simulink model "cf_compare_model"  (R2016a)
settings: Solver=FixedStepAuto  StartTime=0.0  StopTime=50  FixedStep=dt  RelTol=1e-3
values from neighbouring files (symbols this model uses):
  circ_amp = 3    [cf_pid_compare.m]
  circ_w = k    (= 0.666666666667)    [cf_pid_compare.m]
  ic = [-3 0 0 0 0 0 0 0 0 0 0 0]    [cf_pid_compare.m]    (also in main.m = [0 0 0 0 0 0 0 0 0 0 0 0])
  r2d = 180/pi    (= 57.2957795131)    [main.m]
  x_init = 0.0    (= 0)    [cf_pid_compare.m]
  x_vel = 1.0    (= 1)    [cf_pid_compare.m]
undefined symbols (not defined in the file or in its folder): default_ctl, est, geometric_ctl, pid_ctl
undefined symbols (not defined in the file): cf2
libraries: simulink x18, vrlib x12, aerolibtransform2 x12, cstblocks x8, aerolibutil x6, aerolibnav x3, dspmathops x2
(part 1 of 2)
settings Model: Creator=appatte2  LastModifiedBy=arun
settings DebuggingCC: SFUnusedDataAndEventsDiag=none

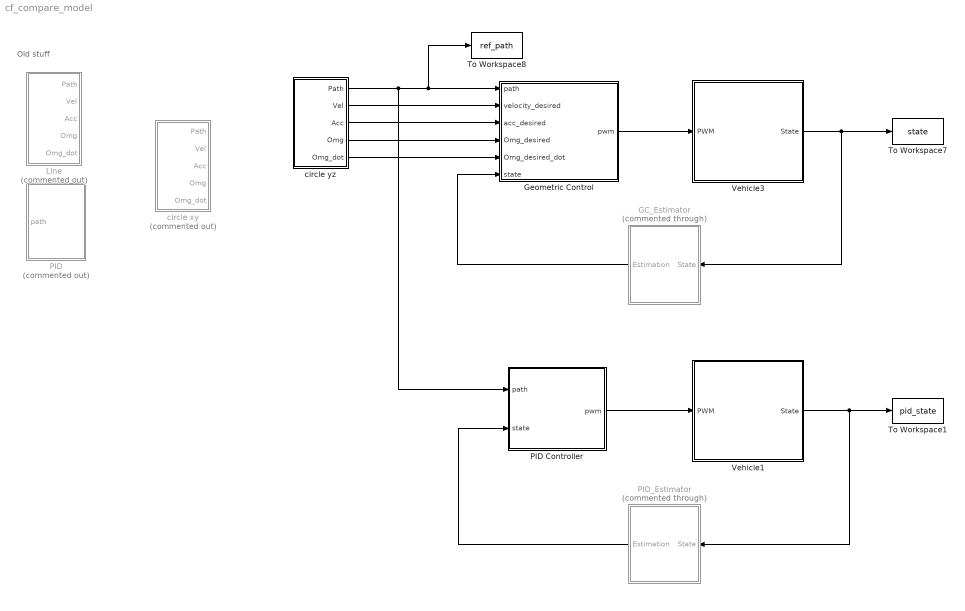
== system cf_compare_model ==
  note: Old stuff
  GC_Estimator : Subsystem  Commented=through  mask{rng_seed=1111, est=est}
      mask prompts: rng_seed "Random Seed"; est "Estimator Params"
  Geometric Control : Subsystem  mask(PID Controller for Quadrotor){model=cf2, ctl=geometric_ctl}
      mask prompts: model "Quad Model"; ctl "Controller"
      mask help: Allows user to set parameters for pid controllers on rates, angles and linear position.
  Line : Subsystem  Commented=on
  PID : Subsystem  Commented=on
  PID Controller : Subsystem  mask(PID Controller for Quadrotor){mix=pid_ctl.mix, rates=pid_ctl.rates, att=pid_ctl.att, pos=pid_ctl.pos, sat=pid_ctl.sat, intSat=pid_ctl.intSat}
      mask prompts: mix "Motor Mixing Table"; rates "Rate Control Table"; att "Attitude Control Table"; pos "Position Control Table"; sat "Attitude Limits"; intSat "Integral Saturation"
      mask help: Allows user to set parameters for pid controllers on rates, angles and linear position.
  PID_Estimator : Subsystem  Commented=through  mask{rng_seed=1111, est=est}
      mask prompts: rng_seed "Random Seed"; est "Estimator Params"
  To Workspace1 : ToWorkspace  VariableName=pid_state  SampleTime=-1
  To Workspace7 : ToWorkspace  VariableName=state  SampleTime=-1
  To Workspace8 : ToWorkspace  VariableName=ref_path  SampleTime=-1
      settings: Save2DSignal=2-D array (concatenate along first dimension)
  Vehicle1 : Subsystem  mask{model=cf2, ic=ic}
      mask prompts: model "Model Object"; ic "Initial Condition"
  Vehicle3 : Subsystem  mask{model=cf2, ic=ic}
      mask prompts: model "Model Object"; ic "Initial Condition"
  circle xy : Subsystem  Commented=on
  "circle yz " : Subsystem
  wires:
  "circle yz "/1(Path) -> PID Controller/1(path), Geometric Control/1(path), To Workspace8/1
  "circle yz "/2(Vel) -> Geometric Control/2(velocity_desired)
  "circle yz "/3(Acc) -> Geometric Control/3("acc_desired ")
  "circle yz "/4(Omg) -> Geometric Control/4(Omg_desired)
  "circle yz "/5(Omg_dot) -> Geometric Control/5(Omg_desired_dot)
  GC_Estimator/1(Estimation) -> Geometric Control/6(state)
  Geometric Control/1(pwm) -> Vehicle3/1(PWM)
  Vehicle3/1(State) -> GC_Estimator/1(State), To Workspace7/1
  PID Controller/1(pwm) -> Vehicle1/1(PWM)
  Vehicle1/1(State) -> PID_Estimator/1(State), To Workspace1/1
  PID_Estimator/1(Estimation) -> PID Controller/2(state)

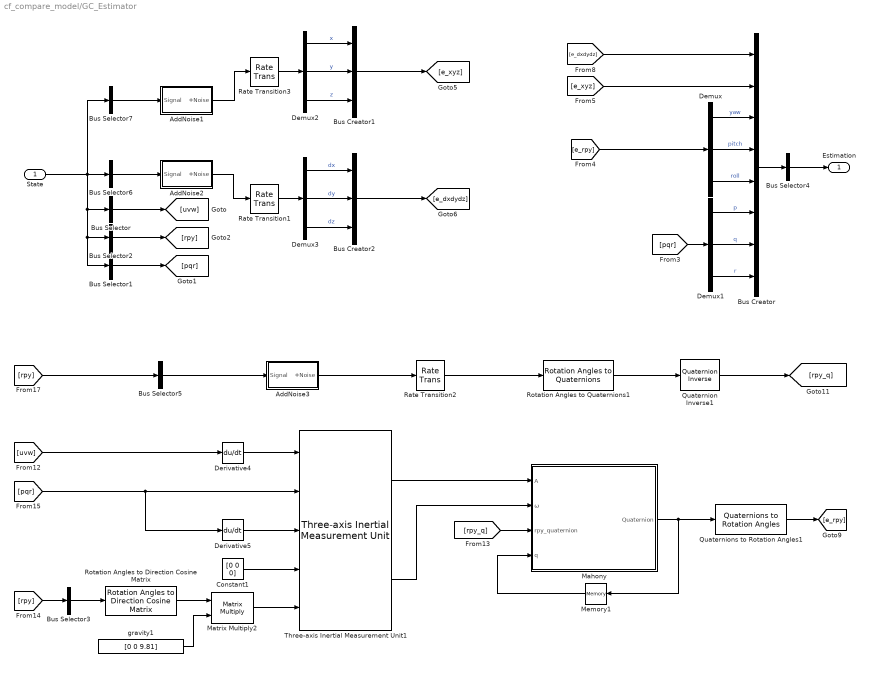
== system cf_compare_model/GC_Estimator ==
  State : Inport
  AddNoise1 : Subsystem
  AddNoise2 : Subsystem
  AddNoise3 : Subsystem
  Bus Creator : BusCreator  Inputs=8
  Bus Creator1 : BusCreator  Inputs=3
  Bus Creator2 : BusCreator  Inputs=3
  Bus Selector : BusSelector  OutputSignals=u,v,w  OutputAsBus=on
  Bus Selector1 : BusSelector  OutputSignals=p,q,r  OutputAsBus=on
  Bus Selector2 : BusSelector  OutputSignals=roll,pitch,yaw  OutputAsBus=on
  Bus Selector3 : BusSelector  OutputSignals=yaw,pitch,roll  OutputAsBus=on
  Bus Selector4 : BusSelector  OutputSignals=signal2.x,signal2.y,signal2.z,signal1.dx,signal1.dy,signal1.dz,roll,pitch,yaw,p,q,r  OutputAsBus=on
  Bus Selector5 : BusSelector  OutputSignals=yaw,pitch,roll  OutputAsBus=on
  Bus Selector6 : BusSelector  OutputSignals=dx,dy,dz  OutputAsBus=on
  Bus Selector7 : BusSelector  OutputSignals=x,y,z  OutputAsBus=on
  Constant1 : Constant  Value=[0 0 0]
  Demux{,1..3} (4 alike) : Demux  Outputs=3
  Derivative4 : Derivative
  Derivative5 : Derivative
  Mahony : Subsystem
  Matrix Multiply2 : Product  Multiplication=Matrix(*)
  Memory1 : Memory  X0=[1 0 0 0]
  Quaternion Inverse1 : aerolibutil/Quaternion Inverse
  Quaternions to Rotation Angles1 : aerolibtransform2/Quaternions to Rotation Angles  rotationOrder=ZYX
  Rate Transition1 : RateTransition  OutPortSampleTime=0.004
  Rate Transition2 : RateTransition  OutPortSampleTime=0.004
  Rate Transition3 : RateTransition  OutPortSampleTime=0.004
  Rotation Angles to Direction Cosine Matrix : aerolibtransform2/Rotation Angles to Direction Cosine Matrix  rotationOrder=ZYX
  Rotation Angles to Quaternions1 : aerolibtransform2/Rotation Angles to Quaternions  rotationOrder=ZYX
  Three-axis Inertial Measurement Unit1 : aerolibnav/Three-axis Inertial Measurement Unit  units=Metric (MKS)  imu=[0 0 0]  dtype_a=on  w_a=190  z_a=0.707  a_sf_cc=[0.98 0 0; 0 0.98 0; 0 0 0.98]  a_bias=[0 0 0]  a_sat="[-19.62  -19.62  -19.62 19.62 19.62 19.62]"  dtype_g=on  w_g=190  z_g=0.707  g_sf_cc=[.98 0 0; 0 .98 0; 0 0 .98]  g_bias=[0 0 0]  g_sens=[0 0 0]  g_sat="[-4.36  -4.36  -4.36 4.36 4.36 4.36]"  i_rand=on  i_seeds=[23093 23094 23095 23096 23097 23098]*rng_seed  i_pow=[0.001 0.001 0.001 0.0001 0.0001 0.0001]*10  i_Ts=0
  gravity1 : Constant  Value=[0 0 9.81]
  Estimation : Outport
  wires:
  Bus Creator2/1 -> [e_dxdydz]
  Demux3/1 -> Bus Creator2/1  "dx"
  Demux3/2 -> Bus Creator2/2  "dy"
  Demux3/3 -> Bus Creator2/3  "dz"
  Bus Creator1/1 -> [e_xyz]
  Demux2/2 -> Bus Creator1/2  "y"
  Demux2/3 -> Bus Creator1/3  "z"
  Demux2/1 -> Bus Creator1/1  "x"
  Bus Selector4/1 -> Estimation/1
  Demux/3 -> Bus Creator/5  "roll"
  Demux/1 -> Bus Creator/3  "yaw"
  Demux/2 -> Bus Creator/4  "pitch"
  Bus Selector2/1 -> [rpy]
  Bus Selector1/1 -> [pqr]
  Bus Selector/1 -> [uvw]
  Bus Creator/1 -> Bus Selector4/1
  State/1 -> Bus Selector6/1, Bus Selector/1, Bus Selector2/1, Bus Selector1/1, Bus Selector7/1
  Demux1/1 -> Bus Creator/6  "p"
  Demux1/2 -> Bus Creator/7  "q"
  [pqr] -> Demux1/1
  Demux1/3 -> Bus Creator/8  "r"
  Quaternions to Rotation Angles1/1 -> [e_rpy]
  [rpy] -> Bus Selector5/1
  AddNoise3/1(+Noise) -> Rate Transition2/1
  Rate Transition2/1 -> Rotation Angles to Quaternions1/1
  [rpy_q] -> Mahony/3(rpy_quaternion)
  Rotation Angles to Quaternions1/1 -> Quaternion Inverse1/1
  [rpy] -> Bus Selector3/1
  [pqr] -> Derivative5/1, Three-axis Inertial Measurement Unit1/2
  [uvw] -> Derivative4/1
  Matrix Multiply2/1 -> Three-axis Inertial Measurement Unit1/5
  Rotation Angles to Direction Cosine Matrix/1 -> Matrix Multiply2/1
  gravity1/1 -> Matrix Multiply2/2
  Derivative5/1 -> Three-axis Inertial Measurement Unit1/3
  Three-axis Inertial Measurement Unit1/2 -> Mahony/2(ω)
  Three-axis Inertial Measurement Unit1/1 -> Mahony/1(A)
  Mahony/1(Quaternion) -> Quaternions to Rotation Angles1/1, Memory1/1
  Memory1/1 -> Mahony/4(q)
  Constant1/1 -> Three-axis Inertial Measurement Unit1/4
  Derivative4/1 -> Three-axis Inertial Measurement Unit1/1
  Bus Selector3/1 -> Rotation Angles to Direction Cosine Matrix/1
  Quaternion Inverse1/1 -> [rpy_q]
  Bus Selector5/1 -> AddNoise3/1(Signal)
  Bus Selector6/1 -> AddNoise2/1(Signal)
  AddNoise1/1(+Noise) -> Rate Transition3/1
  Bus Selector7/1 -> AddNoise1/1(Signal)
  Rate Transition1/1 -> Demux3/1
  Rate Transition3/1 -> Demux2/1
  AddNoise2/1(+Noise) -> Rate Transition1/1
  [e_rpy] -> Demux/1
  [e_dxdydz] -> Bus Creator/1
  [e_xyz] -> Bus Creator/2

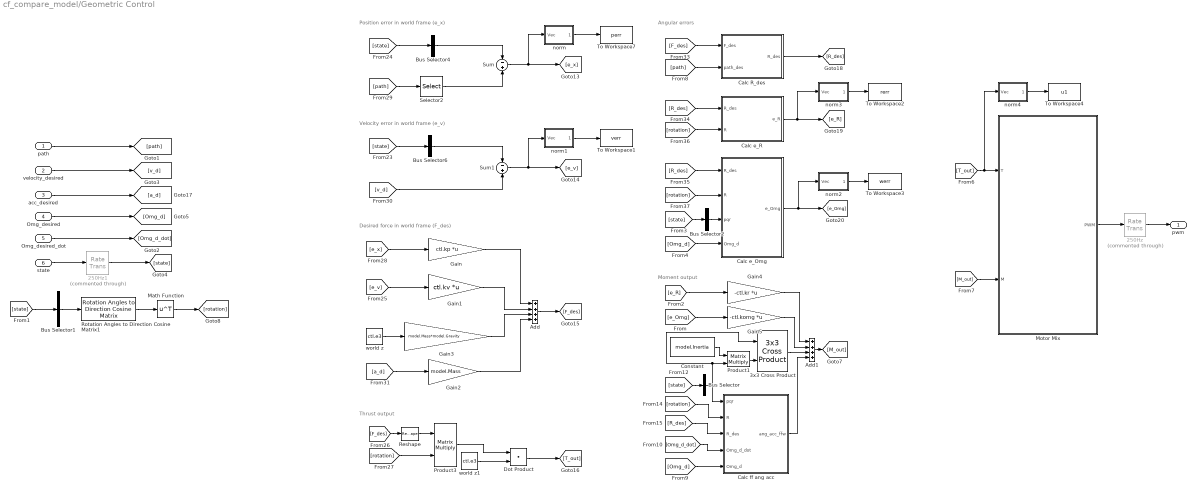
== system cf_compare_model/Geometric Control ==
  note: Moment output
  note: Angular errors
  note: Thrust output
  note: Desired force in world frame (F_des)
  note: Velocity error in world frame (e_v)
  note: Position error in world frame (e_x)
  path : Inport
  velocity_desired : Inport  Port=2
  "acc_desired " : Inport  Port=3
  Omg_desired : Inport  Port=4
  Omg_desired_dot : Inport  Port=5
  state : Inport  Port=6
  250Hz : RateTransition  Commented=through  OutPortSampleTime=0.004
  250Hz1 : RateTransition  Commented=through  OutPortSampleTime=0.004
  3x3 Cross Product : aerolibutil/3x3 Cross Product
  Add : Sum  Inputs=++++
  Add1 : Sum  Inputs=++++
  Bus Selector : BusSelector  OutputSignals=p,q,r  OutputAsBus=on
  Bus Selector1 : BusSelector  OutputSignals=yaw,pitch,roll  OutputAsBus=on
  Bus Selector2 : BusSelector  OutputSignals=p,q,r  OutputAsBus=on
  Bus Selector4 : BusSelector  OutputSignals=x,y,z  OutputAsBus=on
  Bus Selector6 : BusSelector  OutputSignals=dx,dy,dz  OutputAsBus=on
  Calc R_des : Subsystem
  Calc e_Omg : Subsystem
  Calc e_R : Subsystem
  Calc ff ang acc : Subsystem
  Constant : Constant  Value=model.Inertia
  Dot Product : DotProduct  InputSameDT=on  OutDataTypeStr=Inherit: Inherit via internal rule
  Gain : Gain  Gain=ctl.kp  Multiplication=Matrix(K*u) (u vector)
  Gain1 : Gain  Gain=ctl.kv  Multiplication=Matrix(K*u) (u vector)
  Gain2 : Gain  Gain=model.Mass
  Gain3 : Gain  Gain=model.Mass*model.Gravity
  Gain4 : Gain  Gain=-ctl.kr  Multiplication=Matrix(K*u) (u vector)
  Gain5 : Gain  Gain=-ctl.komg  Multiplication=Matrix(K*u) (u vector)
  Math Function : Math  Operator=transpose  SaturateOnIntegerOverflow=on
  Motor Mix : Subsystem
  Product1 : Product  Multiplication=Matrix(*)
  Product3 : Product  Multiplication=Matrix(*)
  Reshape : Reshape  OutputDimensionality=Row vector (2-D)
  Rotation Angles to Direction Cosine Matrix1 : aerolibtransform2/Rotation Angles to Direction Cosine Matrix  rotationOrder=ZYX
  Selector2 : Selector  InputPortWidth=4  IndexOptions=Index vector (dialog)  Indices=[1 2 3]  OutputSizes=1
  Sum : Sum  Inputs=-|+
  Sum1 : Sum  Inputs=-|+
  To Workspace1 : ToWorkspace  VariableName=verr  SaveFormat=Timeseries  SampleTime=-1
  To Workspace2 : ToWorkspace  VariableName=rerr  SaveFormat=Timeseries  SampleTime=-1
  To Workspace3 : ToWorkspace  VariableName=werr  SaveFormat=Timeseries  SampleTime=-1
  To Workspace4 : ToWorkspace  VariableName=u1  SaveFormat=Timeseries  SampleTime=-1
  To Workspace7 : ToWorkspace  VariableName=perr  SaveFormat=Timeseries  SampleTime=-1
  norm : Subsystem
  norm1 : Subsystem
  norm2 : Subsystem
  norm3 : Subsystem
  norm4 : Subsystem
  world z : Constant  Value=ctl.e3
  world z1 : Constant  Value=ctl.e3
  pwm : Outport
  wires:
  state/1 -> 250Hz1/1
  path/1 -> [path]
  velocity_desired/1 -> [v_d]
  Motor Mix/1(PWM) -> 250Hz/1
  [path] -> Selector2/1
  [state] -> Bus Selector4/1
  Bus Selector4/1 -> Sum/1
  [state] -> Bus Selector6/1
  Sum1/1 -> norm1/1(Vec), [e_v]
  [v_d] -> Sum1/2
  [e_x] -> Gain/1
  [e_v] -> Gain1/1
  [a_d] -> Gain2/1
  world z/1 -> Gain3/1
  Gain3/1 -> Add/3
  Gain2/1 -> Add/4
  Gain1/1 -> Add/2
  Gain/1 -> Add/1
  Add/1 -> [F_des]
  [F_des] -> Reshape/1
  Product3/1 -> Dot Product/1
  "acc_desired "/1 -> [a_d]
  [F_des] -> Calc R_des/1(F_des)
  [path] -> Calc R_des/2(path_des)
  Calc R_des/1(R_des) -> [R_des]
  [R_des] -> Calc e_R/1(R_des)
  [rotation] -> Calc e_R/2(R)
  Calc e_R/1(e_R) -> norm3/1(Vec), [e_R]
  [R_des] -> Calc e_Omg/1(R_des)
  [rotation] -> Calc e_Omg/2(R)
  Calc e_Omg/1(e_Omg) -> norm2/1(Vec), [e_Omg]
  Omg_desired/1 -> [Omg_d]
  [state] -> Bus Selector2/1
  [Omg_d] -> Calc e_Omg/4(Omg_d)
  Constant/1 -> Product1/1
  Product1/1 -> 3x3 Cross Product/2
  [e_R] -> Gain4/1
  [e_Omg] -> Gain5/1
  Gain4/1 -> Add1/1
  Gain5/1 -> Add1/2
  [T_out] -> norm4/1(Vec), Motor Mix/1(T)
  [M_out] -> Motor Mix/2(M)
  Sum/1 -> norm/1(Vec), [e_x]
  Selector2/1 -> Sum/2
  Dot Product/1 -> [T_out]
  [rotation] -> Product3/2
  world z1/1 -> Dot Product/2
  Reshape/1 -> Product3/1
  Bus Selector6/1 -> Sum1/1
  Add1/1 -> [M_out]
  Rotation Angles to Direction Cosine Matrix1/1 -> Math Function/1
  Math Function/1 -> [rotation]
  Bus Selector1/1 -> Rotation Angles to Direction Cosine Matrix1/1
  [state] -> Bus Selector1/1
  Omg_desired_dot/1 -> [Omg_d_dot]
  [rotation] -> Calc ff ang acc/2(R)
  [Omg_d_dot] -> Calc ff ang acc/4(Omg_d_dot)
  [Omg_d] -> Calc ff ang acc/5(Omg_d)
  [R_des] -> Calc ff ang acc/3(R_des)
  [state] -> Bus Selector/1
  Bus Selector/1 -> 3x3 Cross Product/1, Product1/2, Calc ff ang acc/1(pqr)
  Bus Selector2/1 -> Calc e_Omg/3(pqr)
  3x3 Cross Product/1 -> Add1/3
  Calc ff ang acc/1(ang_acc_ffw) -> Add1/4
  250Hz/1 -> pwm/1
  250Hz1/1 -> [state]
  norm/1(Norm) -> To Workspace7/1
  norm1/1(Norm) -> To Workspace1/1
  norm2/1(Norm) -> To Workspace3/1
  norm3/1(Norm) -> To Workspace2/1
  norm4/1(Norm) -> To Workspace4/1

== system cf_compare_model/Line ==
  note: X
      | Y
      | Z
      | Yaw
  Constant : Constant  Value=10
  Constant1 : Constant  Commented=on  Value=[2,2,0]'
  Constant2 : Constant  Commented=on  Value=[0,0,0]'
  Constant3 : Constant  Commented=on  Value=[0,0,0]'
  Constant4 : Constant  Commented=on  Value=[0,0,0]'
  Constant5 : Constant  Value=pi/4
  Gain : Gain  Commented=through  Gain=0
  Gain1 : Gain  Commented=through  Gain=0
  Mux : Mux
  Ramp : simulink/Sources/Ramp  slope=2  start=0  X0=0
  Ramp1 : simulink/Sources/Ramp  slope=2  start=0  X0=0
  Path : Outport
  Vel : Outport  Port=2
  Acc : Outport  Port=3
  Omg : Outport  Port=4
  Omg_dot : Outport  Port=5
  wires:
  Mux/1 -> Path/1
  Constant5/1 -> Mux/4
  Constant/1 -> Mux/3
  Ramp/1 -> Gain1/1
  Ramp1/1 -> Gain/1
  Gain/1 -> Mux/2
  Gain1/1 -> Mux/1
  Constant1/1 -> Vel/1
  Constant2/1 -> Acc/1
  Constant3/1 -> Omg/1
  Constant4/1 -> Omg_dot/1

== system cf_compare_model/PID ==
  path : Inport
  Estimator : Subsystem  mask{rng_seed=1111, est=est}
      mask prompts: rng_seed "Random Seed"; est "Estimator params"
  PID Controller : Subsystem  mask(PID Controller for Quadrotor){mix=pid_ctl.mix, rates=pid_ctl.rates, att=pid_ctl.att, pos=pid_ctl.pos, sat=pid_ctl.sat, intSat=pid_ctl.intSat}
      mask prompts: mix "Motor Mixing Table"; rates "Rate Control Table"; att "Attitude Control Table"; pos "Position Control Table"; sat "Attitude Limits"; intSat "Integral Saturation"
      mask help: Allows user to set parameters for pid controllers on rates, angles and linear position.
  To Workspace1 : ToWorkspace  VariableName=pid_state  SampleTime=-1
  Vehicle : Subsystem  mask{model=cf2, ic=ic}
      mask prompts: model "Model Object"; ic "Initial Condition"
  wires:
  path/1 -> PID Controller/1(path)
  PID Controller/1(pwm) -> Vehicle/1(PWM)
  Estimator/1(Estimation) -> PID Controller/2(state)
  Vehicle/1(State) -> Estimator/1(State), To Workspace1/1

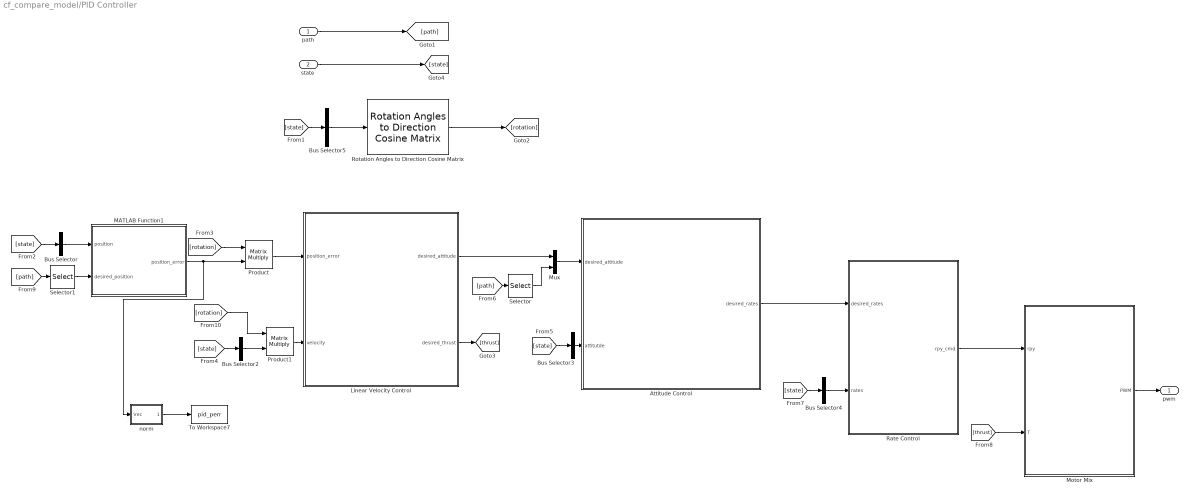
== system cf_compare_model/PID Controller ==
  path : Inport
  state : Inport  Port=2
  Attitude Control : Subsystem
  Bus Selector : BusSelector  OutputSignals=x,y,z  OutputAsBus=on
  Bus Selector2 : BusSelector  OutputSignals=dx,dy,dz  OutputAsBus=on
  Bus Selector3 : BusSelector  OutputSignals=roll,pitch,yaw  OutputAsBus=on
  Bus Selector4 : BusSelector  OutputSignals=p,q,r  OutputAsBus=on
  Bus Selector5 : BusSelector  OutputSignals=yaw,pitch,roll  OutputAsBus=on
  Linear Velocity Control : Subsystem
  MATLAB Function1 : MATLAB Function  TreatAsAtomicUnit=on
  Motor Mix : Subsystem
  Mux : Mux  Inputs=2
  Product : Product  Multiplication=Matrix(*)
  Product1 : Product  Multiplication=Matrix(*)
  Rate Control : Subsystem
  Rotation Angles to Direction Cosine Matrix : aerolibtransform2/Rotation Angles to Direction Cosine Matrix  rotationOrder=ZYX
  Selector : Selector  InputPortWidth=4  IndexOptions=Index vector (dialog)  Indices=[4]  OutputSizes=1
  Selector1 : Selector  InputPortWidth=4  IndexOptions=Index vector (dialog)  Indices=[1 2 3]  OutputSizes=1
  To Workspace7 : ToWorkspace  VariableName=pid_perr  SaveFormat=Timeseries  SampleTime=-1
  norm : Subsystem
  pwm : Outport
  wires:
  [path] -> Selector1/1
  [state] -> Bus Selector/1
  Motor Mix/1(PWM) -> pwm/1
  Selector1/1 -> MATLAB Function1/2(desired_position)
  Bus Selector/1 -> MATLAB Function1/1(position)
  [rotation] -> Product/1
  Mux/1 -> Attitude Control/1(desired_attitude)
  Bus Selector5/1 -> Rotation Angles to Direction Cosine Matrix/1
  [state] -> Bus Selector3/1
  Bus Selector3/1 -> Attitude Control/2(attitutde)
  [state] -> Bus Selector2/1
  [state] -> Bus Selector5/1
  [thrust] -> Motor Mix/2(T)
  Attitude Control/1(desired_rates) -> Rate Control/1(desired_rates)
  [state] -> Bus Selector4/1
  Bus Selector4/1 -> Rate Control/2(rates)
  [path] -> Selector/1
  Selector/1 -> Mux/2
  Linear Velocity Control/2(desired_thrust) -> [thrust]
  state/1 -> [state]
  path/1 -> [path]
  MATLAB Function1/1(position_error) -> norm/1(Vec), Product/2
  Product/1 -> Linear Velocity Control/1(position_error)
  Linear Velocity Control/1(desired_attitude) -> Mux/1
  Rotation Angles to Direction Cosine Matrix/1 -> [rotation]
  Rate Control/1(rpy_cmd) -> Motor Mix/1(rpy)
  Product1/1 -> Linear Velocity Control/2(velocity)
  Bus Selector2/1 -> Product1/2
  [rotation] -> Product1/1
  norm/1(Norm) -> To Workspace7/1

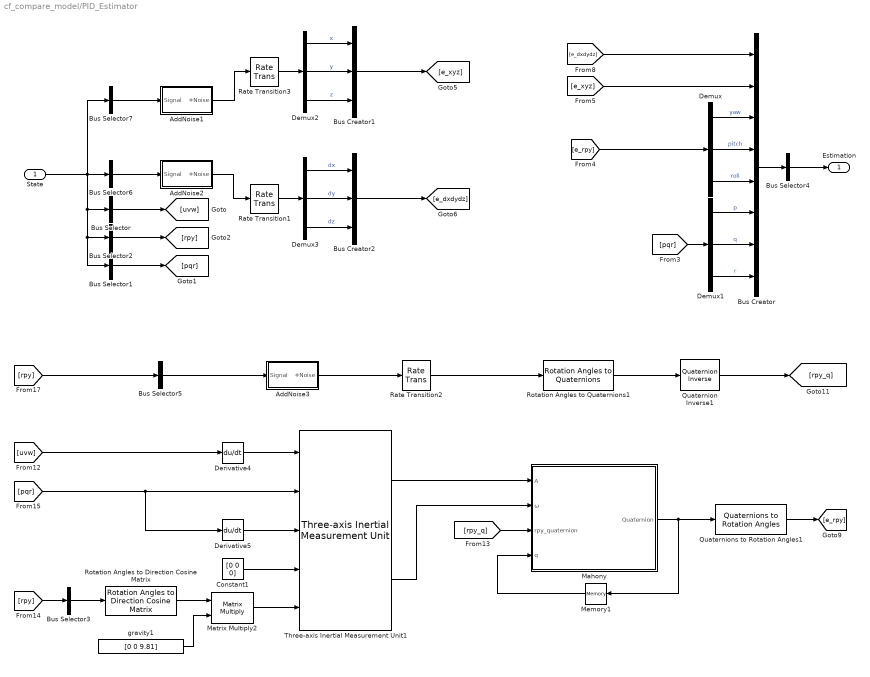
== system cf_compare_model/PID_Estimator ==
  State : Inport
  AddNoise1 : Subsystem
  AddNoise2 : Subsystem
  AddNoise3 : Subsystem
  Bus Creator : BusCreator  Inputs=8
  Bus Creator1 : BusCreator  Inputs=3
  Bus Creator2 : BusCreator  Inputs=3
  Bus Selector : BusSelector  OutputSignals=u,v,w  OutputAsBus=on
  Bus Selector1 : BusSelector  OutputSignals=p,q,r  OutputAsBus=on
  Bus Selector2 : BusSelector  OutputSignals=roll,pitch,yaw  OutputAsBus=on
  Bus Selector3 : BusSelector  OutputSignals=yaw,pitch,roll  OutputAsBus=on
  Bus Selector4 : BusSelector  OutputSignals=signal2.x,signal2.y,signal2.z,signal1.dx,signal1.dy,signal1.dz,roll,pitch,yaw,p,q,r  OutputAsBus=on
  Bus Selector5 : BusSelector  OutputSignals=yaw,pitch,roll  OutputAsBus=on
  Bus Selector6 : BusSelector  OutputSignals=dx,dy,dz  OutputAsBus=on
  Bus Selector7 : BusSelector  OutputSignals=x,y,z  OutputAsBus=on
  Constant1 : Constant  Value=[0 0 0]
  Demux{,1..3} (4 alike) : Demux  Outputs=3
  Derivative4 : Derivative
  Derivative5 : Derivative
  Mahony : Subsystem
  Matrix Multiply2 : Product  Multiplication=Matrix(*)
  Memory1 : Memory  X0=[1 0 0 0]
  Quaternion Inverse1 : aerolibutil/Quaternion Inverse
  Quaternions to Rotation Angles1 : aerolibtransform2/Quaternions to Rotation Angles  rotationOrder=ZYX
  Rate Transition1 : RateTransition  OutPortSampleTime=0.004
  Rate Transition2 : RateTransition  OutPortSampleTime=0.004
  Rate Transition3 : RateTransition  OutPortSampleTime=0.004
  Rotation Angles to Direction Cosine Matrix : aerolibtransform2/Rotation Angles to Direction Cosine Matrix  rotationOrder=ZYX
  Rotation Angles to Quaternions1 : aerolibtransform2/Rotation Angles to Quaternions  rotationOrder=ZYX
  Three-axis Inertial Measurement Unit1 : aerolibnav/Three-axis Inertial Measurement Unit  units=Metric (MKS)  imu=[0 0 0]  dtype_a=on  w_a=190  z_a=0.707  a_sf_cc=[0.98 0 0; 0 0.98 0; 0 0 0.98]  a_bias=[0 0 0]  a_sat="[-19.62  -19.62  -19.62 19.62 19.62 19.62]"  dtype_g=on  w_g=190  z_g=0.707  g_sf_cc=[.98 0 0; 0 .98 0; 0 0 .98]  g_bias=[0 0 0]  g_sens=[0 0 0]  g_sat="[-4.36  -4.36  -4.36 4.36 4.36 4.36]"  i_rand=on  i_seeds=[23093 23094 23095 23096 23097 23098]*rng_seed  i_pow=[0.001 0.001 0.001 0.0001 0.0001 0.0001]*10  i_Ts=0
  gravity1 : Constant  Value=[0 0 9.81]
  Estimation : Outport
  wires:
  Bus Creator2/1 -> [e_dxdydz]
  Demux3/1 -> Bus Creator2/1  "dx"
  Demux3/2 -> Bus Creator2/2  "dy"
  Demux3/3 -> Bus Creator2/3  "dz"
  Bus Creator1/1 -> [e_xyz]
  Demux2/2 -> Bus Creator1/2  "y"
  Demux2/3 -> Bus Creator1/3  "z"
  Demux2/1 -> Bus Creator1/1  "x"
  Bus Selector4/1 -> Estimation/1
  Demux/3 -> Bus Creator/5  "roll"
  Demux/1 -> Bus Creator/3  "yaw"
  Demux/2 -> Bus Creator/4  "pitch"
  Bus Selector2/1 -> [rpy]
  Bus Selector1/1 -> [pqr]
  Bus Selector/1 -> [uvw]
  Bus Creator/1 -> Bus Selector4/1
  State/1 -> Bus Selector6/1, Bus Selector/1, Bus Selector2/1, Bus Selector1/1, Bus Selector7/1
  Demux1/1 -> Bus Creator/6  "p"
  Demux1/2 -> Bus Creator/7  "q"
  [pqr] -> Demux1/1
  Demux1/3 -> Bus Creator/8  "r"
  Quaternions to Rotation Angles1/1 -> [e_rpy]
  [rpy] -> Bus Selector5/1
  AddNoise3/1(+Noise) -> Rate Transition2/1
  Rate Transition2/1 -> Rotation Angles to Quaternions1/1
  [rpy_q] -> Mahony/3(rpy_quaternion)
  Rotation Angles to Quaternions1/1 -> Quaternion Inverse1/1
  [rpy] -> Bus Selector3/1
  [pqr] -> Derivative5/1, Three-axis Inertial Measurement Unit1/2
  [uvw] -> Derivative4/1
  Matrix Multiply2/1 -> Three-axis Inertial Measurement Unit1/5
  Rotation Angles to Direction Cosine Matrix/1 -> Matrix Multiply2/1
  gravity1/1 -> Matrix Multiply2/2
  Derivative5/1 -> Three-axis Inertial Measurement Unit1/3
  Three-axis Inertial Measurement Unit1/2 -> Mahony/2(ω)
  Three-axis Inertial Measurement Unit1/1 -> Mahony/1(A)
  Mahony/1(Quaternion) -> Quaternions to Rotation Angles1/1, Memory1/1
  Memory1/1 -> Mahony/4(q)
  Constant1/1 -> Three-axis Inertial Measurement Unit1/4
  Derivative4/1 -> Three-axis Inertial Measurement Unit1/1
  Bus Selector3/1 -> Rotation Angles to Direction Cosine Matrix/1
  Quaternion Inverse1/1 -> [rpy_q]
  Bus Selector5/1 -> AddNoise3/1(Signal)
  Bus Selector6/1 -> AddNoise2/1(Signal)
  AddNoise1/1(+Noise) -> Rate Transition3/1
  Bus Selector7/1 -> AddNoise1/1(Signal)
  Rate Transition1/1 -> Demux3/1
  Rate Transition3/1 -> Demux2/1
  AddNoise2/1(+Noise) -> Rate Transition1/1
  [e_rpy] -> Demux/1
  [e_dxdydz] -> Bus Creator/1
  [e_xyz] -> Bus Creator/2

== system cf_compare_model/Vehicle1 ==
  PWM : Inport
  PWM 2 Speed : Subsystem
  Vehicle Dynamics : Subsystem
  State : Outport
  wires:
  PWM 2 Speed/1(Omega) -> Vehicle Dynamics/1(Omega)
  PWM/1 -> PWM 2 Speed/1(PWM)
  Vehicle Dynamics/1(State) -> State/1

== system cf_compare_model/Vehicle3 ==
  PWM : Inport
  PWM 2 Speed : Subsystem
  Vehicle Dynamics : Subsystem
  State : Outport
  wires:
  PWM 2 Speed/1(Omega) -> Vehicle Dynamics/1(Omega)
  PWM/1 -> PWM 2 Speed/1(PWM)
  Vehicle Dynamics/1(State) -> State/1

== system cf_compare_model/circle xy ==
  "Calc_Omg_des " : MATLAB Function  TreatAsAtomicUnit=on
  Constant1 : Constant  Value=0
  Constant3 : Constant  Value=0
  Mux : Mux
  Selector{,1..3} (4 alike) : Selector  InputPortWidth=3  IndexOptions=Index vector (dialog)  Indices=[2 3 1]  OutputSizes=1
  Selector4 : Selector  InputPortWidth=4  IndexOptions=Index vector (dialog)  Indices=[2 3 1 4]  OutputSizes=1
  X : simulink/Sources/Ramp  slope=x_vel  start=0  X0=x_init
  Y : Sin  Amplitude=circ_amp  Frequency=circ_w  Phase=pi/2  SampleTime=0
  Yaw : simulink/Sources/Ramp  slope=0  start=0  X0=0
  Z : Sin  Amplitude=circ_amp  Frequency=circ_w  SampleTime=0
  acc_circ : Subsystem
  jerk_circ : Subsystem
  snap_circ : Subsystem
  vel_circ : Subsystem
  Path : Outport
  Vel : Outport  Port=2
  Acc : Outport  Port=3
  Omg : Outport  Port=4
  Omg_dot : Outport  Port=5
  wires:
  Z/1 -> Mux/3
  X/1 -> Mux/1
  Y/1 -> Mux/2
  Yaw/1 -> Mux/4, "Calc_Omg_des "/4(yaw_des)
  Constant3/1 -> "Calc_Omg_des "/5(dyaw_des)
  vel_circ/1(Vel) -> Selector/1
  acc_circ/1(Acc) -> Selector1/1
  jerk_circ/1(Jerk) -> Selector2/1
  "Calc_Omg_des "/1(omg_des) -> Omg/1
  "Calc_Omg_des "/2(omg_des_dot) -> Omg_dot/1
  Constant1/1 -> "Calc_Omg_des "/6(ddyaw_des)
  snap_circ/1(Snap) -> Selector3/1
  Selector/1 -> Vel/1
  Selector1/1 -> "Calc_Omg_des "/1(a_des), Acc/1
  Selector2/1 -> "Calc_Omg_des "/2(j_des)
  Selector3/1 -> "Calc_Omg_des "/3(s_des)
  Mux/1 -> Selector4/1
  Selector4/1 -> Path/1

== system cf_compare_model/circle yz  ==
  "Calc_Omg_des " : MATLAB Function  TreatAsAtomicUnit=on
  Constant1 : Constant  Value=0
  Constant3 : Constant  Value=0
  Mux : Mux
  X : simulink/Sources/Ramp  slope=x_vel  start=0  X0=x_init
  Y : Sin  Amplitude=circ_amp  Frequency=circ_w  Phase=pi/2  SampleTime=0
  Yaw : simulink/Sources/Ramp  slope=0  start=0  X0=0
  Z : Sin  Amplitude=circ_amp  Frequency=circ_w  SampleTime=0
  acc_circ : Subsystem
  jerk_circ : Subsystem
  snap_circ : Subsystem
  vel_circ : Subsystem
  Path : Outport
  Vel : Outport  Port=2
  Acc : Outport  Port=3
  Omg : Outport  Port=4
  Omg_dot : Outport  Port=5
  wires:
  Z/1 -> Mux/3
  X/1 -> Mux/1
  Y/1 -> Mux/2
  Mux/1 -> Path/1
  Yaw/1 -> Mux/4, "Calc_Omg_des "/4(yaw_des)
  Constant3/1 -> "Calc_Omg_des "/5(dyaw_des)
  vel_circ/1(Vel) -> Vel/1
  acc_circ/1(Acc) -> "Calc_Omg_des "/1(a_des), Acc/1
  jerk_circ/1(Jerk) -> "Calc_Omg_des "/2(j_des)
  "Calc_Omg_des "/1(omg_des) -> Omg/1
  "Calc_Omg_des "/2(omg_des_dot) -> Omg_dot/1
  Constant1/1 -> "Calc_Omg_des "/6(ddyaw_des)
  snap_circ/1(Snap) -> "Calc_Omg_des "/3(s_des)

== system cf_compare_model/GC_Estimator/AddNoise1 ==
  Signal : Inport
  Add2 : Sum
  Band-Limited White Noise : simulink/Sources/Band-Limited White Noise  Cov=est.noise_power  Ts=est.noise_sample_time  seed=rng_seed
  +Noise : Outport
  wires:
  Add2/1 -> +Noise/1
  Signal/1 -> Add2/1
  Band-Limited White Noise/1 -> Add2/2

== system cf_compare_model/GC_Estimator/AddNoise2 ==
  Signal : Inport
  Add2 : Sum
  Band-Limited White Noise : simulink/Sources/Band-Limited White Noise  Cov=est.noise_power  Ts=est.noise_sample_time  seed=rng_seed
  +Noise : Outport
  wires:
  Add2/1 -> +Noise/1
  Signal/1 -> Add2/1
  Band-Limited White Noise/1 -> Add2/2

== system cf_compare_model/GC_Estimator/AddNoise3 ==
  Signal : Inport
  Add2 : Sum
  Band-Limited White Noise : simulink/Sources/Band-Limited White Noise  Cov=est.noise_power  Ts=est.noise_sample_time  seed=rng_seed
  +Noise : Outport
  wires:
  Add2/1 -> +Noise/1
  Signal/1 -> Add2/1
  Band-Limited White Noise/1 -> Add2/2

== system cf_compare_model/GC_Estimator/Mahony ==
  A : Inport  PortDimensions=[1 3]
  ω : Inport  Port=2  PortDimensions=[1 3]
  rpy_quaternion : Inport  Port=3
  q : Inport  Port=4  PortDimensions=[1 4]
  Acceleration Error Estimate : Scope  Commented=on
  Add : Sum  Inputs=+++
  Add1 : Sum
  Constant : Constant  Value=0
  Cross Product : vrlib/Utilities/Cross Product
  Cross Product1 : vrlib/Utilities/Cross Product
  Gain1 : Gain  Gain=0.5
  Integrator : Integrator
  Integrator1 : Integrator  InitialCondition=[1,0,0,0]
  Ki : Gain  Gain=est.Ki
  Kp : Gain  Gain=est.Kp
  Mux : Mux  Inputs=2
  Normalize Vector : vrlib/Utilities/Normalize Vector  maxzero=.01
  Normalize Vector1 : vrlib/Utilities/Normalize Vector  maxzero=10e-4
  Total Error Estimate : Scope  Commented=on
  calc v : MATLAB Function  TreatAsAtomicUnit=on
  calc v3 : MATLAB Function  TreatAsAtomicUnit=on
  quatprod : MATLAB Function  TreatAsAtomicUnit=on
  Quaternion : Outport
  wires:
  ω/1 -> Add/3
  Normalize Vector/1 -> Cross Product/2
  calc v3/1(v) -> Cross Product1/1
  Cross Product1/1 -> Add1/1
  rpy_quaternion/1 -> calc v3/1(q)
  Cross Product/1 -> Add1/2, Acceleration Error Estimate/1
  q/1 -> quatprod/1(a), calc v/1(q)
  Normalize Vector1/1 -> Quaternion/1
  Integrator1/1 -> Normalize Vector1/1
  Integrator/1 -> Ki/1
  Mux/1 -> quatprod/2(b)
  quatprod/1(ab) -> Gain1/1
  Gain1/1 -> Integrator1/1
  Kp/1 -> Add/1
  Add/1 -> Mux/2
  calc v/1(v) -> Cross Product1/2, Cross Product/1
  Ki/1 -> Add/2
  Add1/1 -> Total Error Estimate/1, Kp/1, Integrator/1
  Constant/1 -> Mux/1
  A/1 -> Normalize Vector/1

== system cf_compare_model/Geometric Control/Calc R_des ==
  note: y_B,des
  note: x_C,des
  note: z_B,des
  note: x_B,des
  F_des : Inport
  path_des : Inport  Port=2
  3x3 Cross Product : aerolibutil/3x3 Cross Product
  3x3 Cross Product1 : aerolibutil/3x3 Cross Product
  Gain4 : Gain  Gain=0
  Matrix Concatenate : Concatenate  NumInputs=3  Mode=Multidimensional array  ConcatenateDimension=2
  Mux : Mux  Inputs=3
  Normalization : dspmathops/Normalization  NormType=2-norm  Bias=1e-10  NormOver=Each column  Dimension=1  outputDataTypeStr=Inherit: Same as product output  outputLastDataTypeStr=Inherit: Same as product output  outputMin=[]  outputMax=[]  accumDataTypeStr=Inherit: Same as product output  accumLastDataTypeStr=Inherit: Same as product output  roundingMode=Floor  overflowMode=off
  Normalization1 : dspmathops/Normalization  NormType=2-norm  Bias=1e-10  NormOver=Each column  Dimension=1  outputDataTypeStr=Inherit: Same as product output  outputLastDataTypeStr=Inherit: Same as product output  outputMin=[]  outputMax=[]  accumDataTypeStr=Inherit: Same as product output  accumLastDataTypeStr=Inherit: Same as product output  roundingMode=Floor  overflowMode=off
  Trigonometric Function : Trigonometry
  Trigonometric Function1 : Trigonometry  Operator=cos
  phi_des : Selector  InputPortWidth=4  IndexOptions=Index vector (dialog)  Indices=[4]  OutputSizes=1
  R_des : Outport
  wires:
  3x3 Cross Product1/1 -> Matrix Concatenate/1
  F_des/1 -> Normalization/1
  path_des/1 -> phi_des/1
  Gain4/1 -> Mux/3
  Trigonometric Function1/1 -> Mux/1
  3x3 Cross Product/1 -> Normalization1/1
  Normalization1/1 -> 3x3 Cross Product1/1, Matrix Concatenate/2
  Trigonometric Function/1 -> Mux/2
  Normalization/1 -> 3x3 Cross Product/1, Matrix Concatenate/3, 3x3 Cross Product1/2
  Mux/1 -> 3x3 Cross Product/2
  phi_des/1 -> Gain4/1, Trigonometric Function/1, Trigonometric Function1/1
  Matrix Concatenate/1 -> R_des/1

== system cf_compare_model/Geometric Control/Calc e_Omg ==
  R_des : Inport
  R : Inport  Port=2
  pqr : Inport  Port=3
  Omg_d : Inport  Port=4
  Math Function2 : Math  Operator=transpose  SaturateOnIntegerOverflow=on
  Product2 : Product  Multiplication=Matrix(*)
  Product3 : Product  Multiplication=Matrix(*)
  Subtract : Sum  Inputs=+-
  e_Omg : Outport
  wires:
  Math Function2/1 -> Product2/1
  R/1 -> Math Function2/1
  Product2/1 -> Product3/1
  R_des/1 -> Product2/2
  Subtract/1 -> e_Omg/1
  pqr/1 -> Subtract/1
  Product3/1 -> Subtract/2
  Omg_d/1 -> Product3/2

== system cf_compare_model/Geometric Control/Calc e_R ==
  R_des : Inport
  R : Inport  Port=2
  Constant : Constant  Commented=on
  Demux : Demux  Outputs=3
  Divide : Product  Commented=on  Inputs=/*
  Gain1 : Gain  Gain=-1
  Gain4 : Gain  Gain=0.5
  Math Function1 : Math  Operator=transpose  SaturateOnIntegerOverflow=on
  Math Function2 : Math  Operator=transpose  SaturateOnIntegerOverflow=on
  Mux : Mux  Inputs=3
  Product : Product  Multiplication=Matrix(*)
  Product1 : Product  Multiplication=Matrix(*)
  Reshape : Reshape
  Reshape1 : Reshape  Commented=on
  Scope1 : Scope  Commented=on
  Scope2 : Scope  Commented=on
  Sqrt : Sqrt  Commented=on  SaturateOnIntegerOverflow=on
  Sum : Sum  Commented=on  Inputs=++|
  Sum of Elements : Sum  Commented=on  Inputs=+
  Sum3 : Sum  Inputs=+|-
  trace elem : Selector  Commented=on  InputPortWidth=9  IndexOptions=Index vector (dialog)  Indices=[1 5 9]  OutputSizes=1
  vee map : Selector  InputPortWidth=9  IndexOptions=Index vector (dialog)  Indices=[2 3 6]  OutputSizes=1
  e_R : Outport
  wires:
  Math Function2/1 -> Product1/1
  Sum3/1 -> Gain4/1
  Product/1 -> Reshape1/1, Sum3/1
  R/1 -> Product/2, Math Function2/1
  Product1/1 -> Sum3/2
  Math Function1/1 -> Product/1
  vee map/1 -> Demux/1
  Gain4/1 -> Reshape/1
  Reshape/1 -> vee map/1
  R_des/1 -> Product1/2, Math Function1/1
  Demux/1 -> Mux/3
  Demux/3 -> Mux/1
  Gain1/1 -> Mux/2
  Demux/2 -> Gain1/1
  Reshape1/1 -> trace elem/1
  trace elem/1 -> Sum of Elements/1
  Sum of Elements/1 -> Sum/2
  Constant/1 -> Sum/1
  Sum/1 -> Scope1/1, Sqrt/1
  Sqrt/1 -> Divide/1, Scope2/1
  Mux/1 -> e_R/1

== system cf_compare_model/Geometric Control/Calc ff ang acc ==
  pqr : Inport
  R : Inport  Port=2
  R_des : Inport  Port=3
  Omg_d_dot : Inport  Port=4
  Omg_d : Inport  Port=5
  Bus Selector : BusSelector  OutputSignals=p,q,r
  Constant : Constant  Value=0
  Constant1 : Constant  Value=0
  Constant2 : Constant  Value=0
  Constant3 : Constant  Value=model.Inertia
  Gain : Gain  Gain=-1
  Gain1 : Gain  Gain=-1
  Gain2 : Gain  Gain=-1
  Math Function : Math  Operator=transpose  SaturateOnIntegerOverflow=on
  Matrix Multiply{,1..4} (5 alike) : Product  Multiplication=Matrix(*)
  Product1 : Product  Multiplication=Matrix(*)
  Sum : Sum  Inputs=+|-
  hat map : aerolibutil/Create 3x3 Matrix
  ang_acc_ffw : Outport
  wires:
  pqr/1 -> Bus Selector/1
  Gain/1 -> hat map/2
  Gain1/1 -> hat map/6
  Gain2/1 -> hat map/7
  Bus Selector/3 -> hat map/4, Gain/1  "<r>"
  Bus Selector/2 -> hat map/3, Gain2/1  "<q>"
  Constant/1 -> hat map/1
  Bus Selector/1 -> hat map/8, Gain1/1  "<p>"
  Constant1/1 -> hat map/5
  Constant2/1 -> hat map/9
  hat map/1 -> Matrix Multiply/1
  R/1 -> Math Function/1
  Math Function/1 -> Matrix Multiply3/1, Matrix Multiply/2
  Matrix Multiply/1 -> Matrix Multiply1/1
  R_des/1 -> Matrix Multiply3/2, Matrix Multiply1/2
  Matrix Multiply1/1 -> Matrix Multiply2/1
  Omg_d/1 -> Matrix Multiply2/2
  Matrix Multiply3/1 -> Matrix Multiply4/1
  Omg_d_dot/1 -> Matrix Multiply4/2
  Matrix Multiply2/1 -> Sum/1
  Matrix Multiply4/1 -> Sum/2
  Sum/1 -> Product1/2
  Product1/1 -> ang_acc_ffw/1
  Constant3/1 -> Product1/1

== system cf_compare_model/Geometric Control/Motor Mix ==
  T : Inport
  M : Inport  Port=2
  Constant : Constant  Value=geometric_ctl.mix
  Demux : Demux  Outputs=3
  Gain1 : Gain  Gain=ctl.thrust_gain
  Gain2 : Gain  Gain=ctl.moment_gain
  Mux : Mux
  Product : Product  Multiplication=Matrix(*)
  Saturation1 : Saturate  UpperLimit=ctl.sat(3,1)  LowerLimit=0
  Saturation3 : Saturate  UpperLimit=ctl.sat(1,1)  LowerLimit=ctl.sat(2,1)
  PWM : Outport
  wires:
  Mux/1 -> Product/2
  Constant/1 -> Product/1
  M/1 -> Gain2/1
  Product/1 -> PWM/1
  Demux/2 -> Mux/2
  Demux/1 -> Mux/1
  Demux/3 -> Mux/3
  Gain1/1 -> Saturation1/1
  T/1 -> Gain1/1
  Gain2/1 -> Saturation3/1
  Saturation3/1 -> Demux/1
  Saturation1/1 -> Mux/4

== system cf_compare_model/Geometric Control/norm ==
  Vec : Inport
  Dot Product1 : DotProduct  InputSameDT=on  OutDataTypeStr=Inherit: Inherit via internal rule
  Math Function1 : Math  Operator=transpose  SaturateOnIntegerOverflow=on
  Sqrt : Sqrt  SaturateOnIntegerOverflow=on
  Norm : Outport
  wires:
  Vec/1 -> Math Function1/1, Dot Product1/1
  Dot Product1/1 -> Sqrt/1
  Math Function1/1 -> Dot Product1/2
  Sqrt/1 -> Norm/1

== system cf_compare_model/Geometric Control/norm1 ==
  Vec : Inport
  Dot Product1 : DotProduct  InputSameDT=on  OutDataTypeStr=Inherit: Inherit via internal rule
  Math Function1 : Math  Operator=transpose  SaturateOnIntegerOverflow=on
  Sqrt : Sqrt  SaturateOnIntegerOverflow=on
  Norm : Outport
  wires:
  Vec/1 -> Math Function1/1, Dot Product1/1
  Dot Product1/1 -> Sqrt/1
  Math Function1/1 -> Dot Product1/2
  Sqrt/1 -> Norm/1

== system cf_compare_model/Geometric Control/norm2 ==
  Vec : Inport
  Dot Product1 : DotProduct  InputSameDT=on  OutDataTypeStr=Inherit: Inherit via internal rule
  Math Function1 : Math  Operator=transpose  SaturateOnIntegerOverflow=on
  Sqrt : Sqrt  SaturateOnIntegerOverflow=on
  Norm : Outport
  wires:
  Vec/1 -> Math Function1/1, Dot Product1/1
  Dot Product1/1 -> Sqrt/1
  Math Function1/1 -> Dot Product1/2
  Sqrt/1 -> Norm/1

== system cf_compare_model/Geometric Control/norm3 ==
  Vec : Inport
  Dot Product1 : DotProduct  InputSameDT=on  OutDataTypeStr=Inherit: Inherit via internal rule
  Math Function1 : Math  Operator=transpose  SaturateOnIntegerOverflow=on
  Sqrt : Sqrt  SaturateOnIntegerOverflow=on
  Norm : Outport
  wires:
  Vec/1 -> Math Function1/1, Dot Product1/1
  Dot Product1/1 -> Sqrt/1
  Math Function1/1 -> Dot Product1/2
  Sqrt/1 -> Norm/1

== system cf_compare_model/Geometric Control/norm4 ==
  Vec : Inport
  Dot Product1 : DotProduct  InputSameDT=on  OutDataTypeStr=Inherit: Inherit via internal rule
  Math Function1 : Math  Operator=transpose  SaturateOnIntegerOverflow=on
  Sqrt : Sqrt  SaturateOnIntegerOverflow=on
  Norm : Outport
  wires:
  Vec/1 -> Math Function1/1, Dot Product1/1
  Dot Product1/1 -> Sqrt/1
  Math Function1/1 -> Dot Product1/2
  Sqrt/1 -> Norm/1

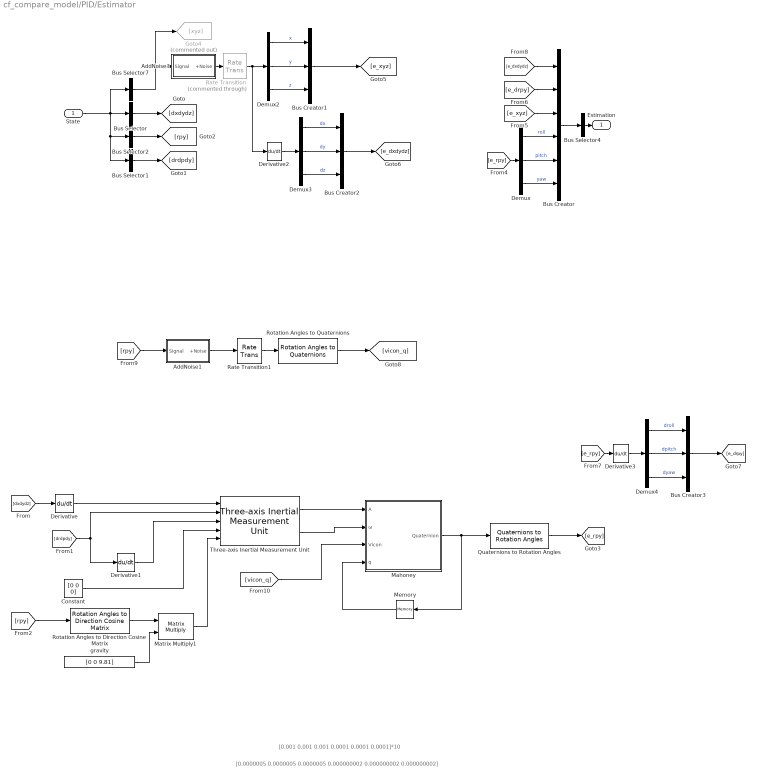
== system cf_compare_model/PID/Estimator ==
  note: [0.001 0.001 0.001 0.0001 0.0001 0.0001]*10
  note: [0.0000005 0.0000005 0.0000005 0.000000002 0.000000002 0.000000002]
  State : Inport
  AddNoise1 : Subsystem
  AddNoise3 : Subsystem
  Bus Creator : BusCreator  Inputs=6
  Bus Creator1 : BusCreator  Inputs=3
  Bus Creator2 : BusCreator  Inputs=3
  Bus Creator3 : BusCreator  Inputs=3
  Bus Selector : BusSelector  OutputSignals=dx,dy,dz  OutputAsBus=on
  Bus Selector1 : BusSelector  OutputSignals=droll,dpitch,dyaw  OutputAsBus=on
  Bus Selector2 : BusSelector  OutputSignals=roll,pitch,yaw  OutputAsBus=on
  Bus Selector4 : BusSelector  OutputSignals=roll,pitch,yaw,signal3.x,signal3.y,signal3.z,signal2.droll,signal2.dpitch,signal2.dyaw,signal1.dx,signal1.dy,signal1.dz  OutputAsBus=on
  Bus Selector7 : BusSelector  OutputSignals=x,y,z  OutputAsBus=on
  Constant : Constant  Value=[0 0 0]
  Demux{,2..4} (4 alike) : Demux  Outputs=3
  Derivative{,1..3} (4 alike) : Derivative
  Goto4 : Goto  Commented=on  GotoTag=xyz
  Mahoney : Subsystem
  Matrix Multiply1 : Product  Multiplication=Matrix(*)
  Memory : Memory  X0=[1 0 0 0]
  Quaternions to Rotation Angles : aerolibtransform2/Quaternions to Rotation Angles  rotationOrder=XYZ
  Rate Transition : RateTransition  Commented=through  OutPortSampleTime=0.005
  Rate Transition1 : RateTransition  OutPortSampleTime=0.005
  Rotation Angles to Direction Cosine Matrix : aerolibtransform2/Rotation Angles to Direction Cosine Matrix  rotationOrder=XYZ
  Rotation Angles to Quaternions : aerolibtransform2/Rotation Angles to Quaternions  rotationOrder=XYZ
  Three-axis Inertial Measurement Unit : aerolibnav/Three-axis Inertial Measurement Unit  units=Metric (MKS)  imu=[0 0 0]  dtype_a=on  w_a=190  z_a=0.707  a_sf_cc=[0.98 0 0; 0 0.98 0; 0 0 0.98]  a_bias=[0 0 0]  a_sat="[-19.62  -19.62  -19.62 19.62 19.62 19.62]"  dtype_g=on  w_g=190  z_g=0.707  g_sf_cc=[.98 0 0; 0 .98 0; 0 0 .98]  g_bias=[0 0 0]  g_sens=[0 0 0]  g_sat="[-4.36  -4.36  -4.36 4.36 4.36 4.36]"  i_rand=on  i_seeds=[23093 23094 23095 23096 23097 23098]*rng_seed  i_pow=[0.001 0.001 0.001 0.0001 0.0001 0.0001]*10  i_Ts=0
  gravity : Constant  Value=[0 0 9.81]
  Estimation : Outport
  wires:
  State/1 -> Bus Selector1/1, Bus Selector2/1, Bus Selector7/1, Bus Selector/1
  Bus Creator/1 -> Bus Selector4/1
  Derivative/1 -> Three-axis Inertial Measurement Unit/1
  Constant/1 -> Three-axis Inertial Measurement Unit/4
  Memory/1 -> Mahoney/4(q)
  Mahoney/1(Quaternion) -> Memory/1, Quaternions to Rotation Angles/1
  Three-axis Inertial Measurement Unit/1 -> Mahoney/1(A)
  Three-axis Inertial Measurement Unit/2 -> Mahoney/2(ω)
  Derivative1/1 -> Three-axis Inertial Measurement Unit/3
  gravity/1 -> Matrix Multiply1/2
  Rotation Angles to Direction Cosine Matrix/1 -> Matrix Multiply1/1
  Matrix Multiply1/1 -> Three-axis Inertial Measurement Unit/5
  Bus Selector/1 -> [dxdydz]
  [dxdydz] -> Derivative/1
  Bus Selector1/1 -> [drdpdy]
  [drdpdy] -> Three-axis Inertial Measurement Unit/2, Derivative1/1
  Bus Selector2/1 -> [rpy]
  [rpy] -> Rotation Angles to Direction Cosine Matrix/1
  Demux/2 -> Bus Creator/5  "pitch"
  Demux/1 -> Bus Creator/4  "roll"
  [e_rpy] -> Demux/1
  Demux/3 -> Bus Creator/6  "yaw"
  Bus Selector4/1 -> Estimation/1
  [e_xyz] -> Bus Creator/3
  [e_drpy] -> Bus Creator/2
  [e_dxdydz] -> Bus Creator/1
  Bus Selector7/1 -> Goto4/1, AddNoise3/1(Signal)
  AddNoise3/1(+Noise) -> Rate Transition/1
  Rate Transition/1 -> Derivative2/1, Demux2/1
  Demux2/1 -> Bus Creator1/1  "x"
  Demux2/3 -> Bus Creator1/3  "z"
  Demux2/2 -> Bus Creator1/2  "y"
  Bus Creator1/1 -> [e_xyz]
  Demux3/3 -> Bus Creator2/3  "dz"
  Derivative2/1 -> Demux3/1
  Demux3/2 -> Bus Creator2/2  "dy"
  Demux3/1 -> Bus Creator2/1  "dx"
  Bus Creator2/1 -> [e_dxdydz]
  Demux4/3 -> Bus Creator3/3  "dyaw"
  Derivative3/1 -> Demux4/1
  Demux4/2 -> Bus Creator3/2  "dpitch"
  Demux4/1 -> Bus Creator3/1  "droll"
  Bus Creator3/1 -> [e_drpy]
  [e_rpy] -> Derivative3/1
  Rotation Angles to Quaternions/1 -> [vicon_q]
  [vicon_q] -> Mahoney/3(Vicon)
  Rate Transition1/1 -> Rotation Angles to Quaternions/1
  AddNoise1/1(+Noise) -> Rate Transition1/1
  [rpy] -> AddNoise1/1(Signal)
  Quaternions to Rotation Angles/1 -> [e_rpy]

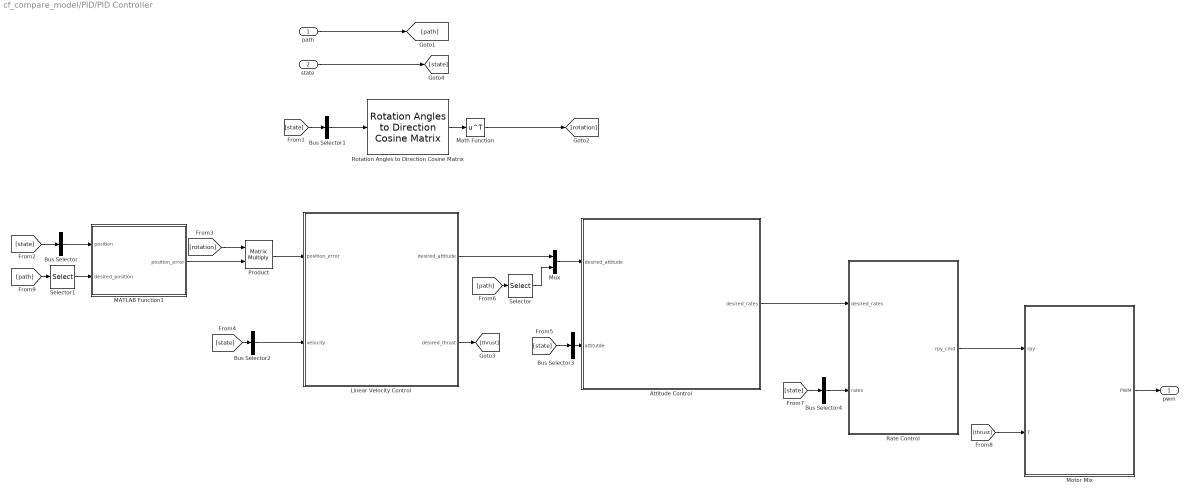
== system cf_compare_model/PID/PID Controller ==
  path : Inport
  state : Inport  Port=2
  Attitude Control : Subsystem
  Bus Selector : BusSelector  OutputSignals=x,y,z  OutputAsBus=on
  Bus Selector1 : BusSelector  OutputSignals=roll,pitch,yaw  OutputAsBus=on
  Bus Selector2 : BusSelector  OutputSignals=dx,dy,dz  OutputAsBus=on
  Bus Selector3 : BusSelector  OutputSignals=roll,pitch,yaw  OutputAsBus=on
  Bus Selector4 : BusSelector  OutputSignals=droll,dpitch,dyaw  OutputAsBus=on
  Linear Velocity Control : Subsystem
  MATLAB Function1 : MATLAB Function  TreatAsAtomicUnit=on
  Math Function : Math  Operator=transpose  SaturateOnIntegerOverflow=on
  Motor Mix : Subsystem
  Mux : Mux  Inputs=2
  Product : Product  Multiplication=Matrix(*)
  Rate Control : Subsystem
  Rotation Angles to Direction Cosine Matrix : aerolibtransform2/Rotation Angles to Direction Cosine Matrix  rotationOrder=ZYX
  Selector : Selector  InputPortWidth=4  IndexOptions=Index vector (dialog)  Indices=[4]  OutputSizes=1
  Selector1 : Selector  InputPortWidth=4  IndexOptions=Index vector (dialog)  Indices=[1 2 3]  OutputSizes=1
  pwm : Outport
  wires:
  [path] -> Selector1/1
  [state] -> Bus Selector/1
  Motor Mix/1(PWM) -> pwm/1
  Selector1/1 -> MATLAB Function1/2(desired_position)
  Bus Selector/1 -> MATLAB Function1/1(position)
  [rotation] -> Product/1
  Mux/1 -> Attitude Control/1(desired_attitude)
  Bus Selector1/1 -> Rotation Angles to Direction Cosine Matrix/1
  [state] -> Bus Selector3/1
  Bus Selector3/1 -> Attitude Control/2(attitutde)
  [state] -> Bus Selector2/1
  [state] -> Bus Selector1/1
  [thrust] -> Motor Mix/2(T)
  Attitude Control/1(desired_rates) -> Rate Control/1(desired_rates)
  [state] -> Bus Selector4/1
  Bus Selector4/1 -> Rate Control/2(rates)
  [path] -> Selector/1
  Selector/1 -> Mux/2
  Linear Velocity Control/2(desired_thrust) -> [thrust]
  state/1 -> [state]
  path/1 -> [path]
  MATLAB Function1/1(position_error) -> Product/2
  Rotation Angles to Direction Cosine Matrix/1 -> Math Function/1
  Product/1 -> Linear Velocity Control/1(position_error)
  Linear Velocity Control/1(desired_attitude) -> Mux/1
  Math Function/1 -> [rotation]
  Rate Control/1(rpy_cmd) -> Motor Mix/1(rpy)
  Bus Selector2/1 -> Linear Velocity Control/2(velocity)

== system cf_compare_model/PID/Vehicle ==
  PWM : Inport
  PWM 2 Speed : Subsystem
  Vehicle Dynamics : Subsystem
  State : Outport
  wires:
  Vehicle Dynamics/1(State) -> State/1
  PWM/1 -> PWM 2 Speed/1(PWM)
  PWM 2 Speed/1(Omega) -> Vehicle Dynamics/1(Omega)

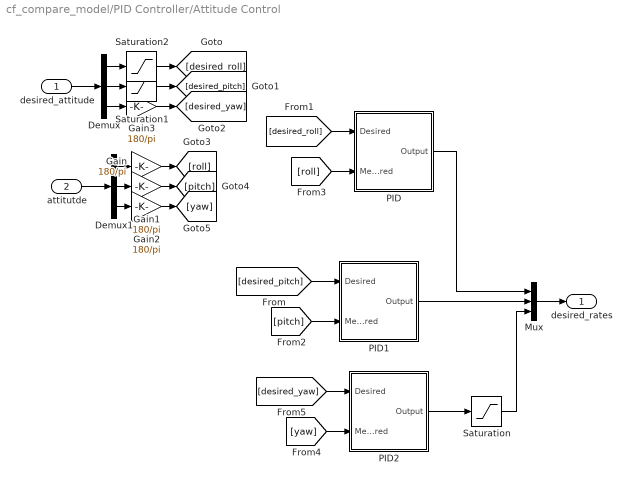
== system cf_compare_model/PID Controller/Attitude Control ==
  desired_attitude : Inport
  attitutde : Inport  Port=2
  Demux : Demux  Outputs=3
  Demux1 : Demux  Outputs=3
  Gain{,1..3} (4 alike) : Gain  Gain=180/pi
  Mux : Mux  Inputs=3
  PID : Subsystem
  PID1 : Subsystem
  PID2 : Subsystem
  Saturation : Saturate  UpperLimit=sat(3)  LowerLimit=-sat(3)
  Saturation1 : Saturate  UpperLimit=sat(2)  LowerLimit=-sat(2)
  Saturation2 : Saturate  UpperLimit=sat(1)  LowerLimit=-sat(1)
  desired_rates : Outport
  wires:
  [pitch] -> PID1/2(Measured)
  [desired_pitch] -> PID1/1(Desired)
  [desired_roll] -> PID/1(Desired)
  [roll] -> PID/2(Measured)
  desired_attitude/1 -> Demux/1
  Demux/1 -> Saturation2/1
  Demux/2 -> Saturation1/1
  Demux/3 -> Gain3/1
  attitutde/1 -> Demux1/1
  Demux1/1 -> Gain/1
  Demux1/2 -> Gain1/1
  Demux1/3 -> Gain2/1
  [yaw] -> PID2/2(Measured)
  Gain/1 -> [roll]
  Gain1/1 -> [pitch]
  Gain2/1 -> [yaw]
  [desired_yaw] -> PID2/1(Desired)
  PID/1(Output) -> Mux/1
  PID2/1(Output) -> Saturation/1
  PID1/1(Output) -> Mux/2
  Mux/1 -> desired_rates/1
  Saturation/1 -> Mux/3
  Saturation1/1 -> [desired_pitch]
  Saturation2/1 -> [desired_roll]
  Gain3/1 -> [desired_yaw]

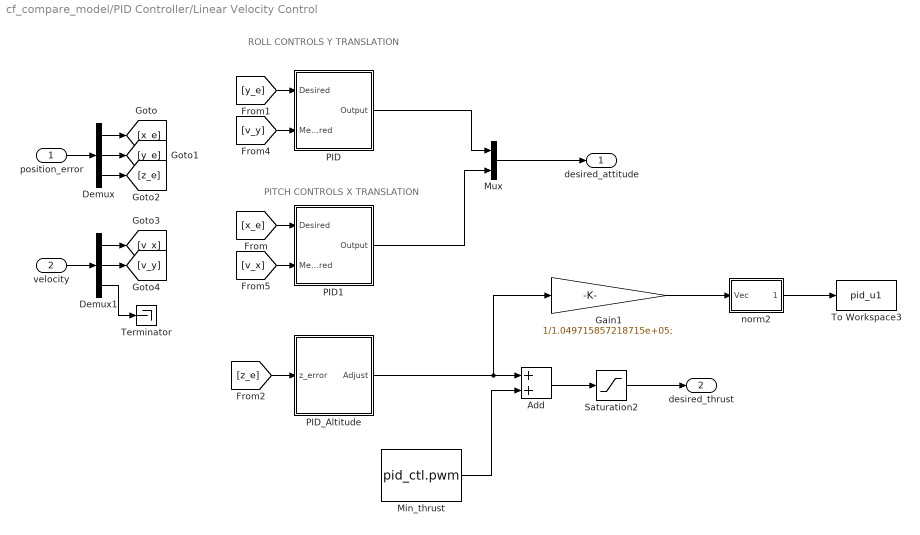
== system cf_compare_model/PID Controller/Linear Velocity Control ==
  note: ROLL CONTROLS Y TRANSLATION
  note: PITCH CONTROLS X TRANSLATION
  position_error : Inport
  velocity : Inport  Port=2
  Add : Sum
  Demux : Demux  Outputs=3
  Demux1 : Demux  Outputs=3
  Gain1 : Gain  Gain=1/1.049715857218715e+05;
  "Min_thrust " : Constant  Value=pid_ctl.pwm  SampleTime=0
  Mux : Mux  Inputs=2
  PID : Subsystem
  PID1 : Subsystem
  PID_Altitude : Subsystem
  Saturation2 : Saturate  UpperLimit=sat(4)  LowerLimit=0
  Terminator : Terminator
  To Workspace3 : ToWorkspace  VariableName=pid_u1  SaveFormat=Timeseries  SampleTime=-1
  norm2 : Subsystem
  desired_attitude : Outport
  desired_thrust : Outport  Port=2
  wires:
  [y_e] -> PID/1(Desired)
  Saturation2/1 -> desired_thrust/1
  "Min_thrust "/1 -> Add/2
  Add/1 -> Saturation2/1
  PID_Altitude/1(Adjust) -> Gain1/1, Add/1
  position_error/1 -> Demux/1
  Demux/1 -> [x_e]
  Demux/2 -> [y_e]
  Demux/3 -> [z_e]
  [z_e] -> PID_Altitude/1(z_error)
  velocity/1 -> Demux1/1
  Demux1/1 -> [v_x]
  Demux1/2 -> [v_y]
  Demux1/3 -> Terminator/1
  [v_y] -> PID/2(Measured)
  Mux/1 -> desired_attitude/1
  PID/1(Output) -> Mux/1
  [x_e] -> PID1/1(Desired)
  [v_x] -> PID1/2(Measured)
  PID1/1(Output) -> Mux/2
  norm2/1(Norm) -> To Workspace3/1
  Gain1/1 -> norm2/1(Vec)

== system cf_compare_model/PID Controller/Motor Mix ==
  rpy : Inport
  T : Inport  Port=2
  Constant : Constant  Value=mix
  Demux : Demux  Outputs=3
  Mux : Mux
  Product : Product  Multiplication=Matrix(*)
  PWM : Outport
  wires:
  T/1 -> Mux/4
  Mux/1 -> Product/2
  Product/1 -> PWM/1
  Constant/1 -> Product/1
  Demux/2 -> Mux/2
  Demux/1 -> Mux/1
  Demux/3 -> Mux/3
  rpy/1 -> Demux/1

== system cf_compare_model/PID Controller/Rate Control ==
  note: roll
      | pitch
      | yaw
  desired_rates : Inport
  rates : Inport  Port=2
  Demux : Demux  Outputs=3
  Demux1 : Demux  Outputs=3
  Gain3 : Gain  Gain=180/pi
  Gain4 : Gain  Gain=180/pi
  Gain5 : Gain  Gain=180/pi
  Mux : Mux  Inputs=3
  PID : Subsystem
  PID1 : Subsystem
  PID2 : Subsystem
  rpy_cmd : Outport
  wires:
  desired_rates/1 -> Demux/1
  Demux/1 -> [desired_droll]
  Demux/2 -> [desired_dpitch]
  Demux/3 -> [desired_dyaw]
  rates/1 -> Demux1/1
  Demux1/1 -> Gain3/1
  Demux1/2 -> Gain4/1
  Demux1/3 -> Gain5/1
  Gain3/1 -> [droll]
  Gain4/1 -> [dpitch]
  Gain5/1 -> [dyaw]
  PID2/1(Output) -> Mux/3
  PID1/1(Output) -> Mux/2
  PID/1(Output) -> Mux/1
  Mux/1 -> rpy_cmd/1
  [desired_dyaw] -> PID2/1(Desired)
  [desired_droll] -> PID/1(Desired)
  [desired_dpitch] -> PID1/1(Desired)
  [dpitch] -> PID1/2(Measured)
  [droll] -> PID/2(Measured)
  [dyaw] -> PID2/2(Measured)

== system cf_compare_model/PID Controller/norm ==
  Vec : Inport
  Dot Product1 : DotProduct  InputSameDT=on  OutDataTypeStr=Inherit: Inherit via internal rule
  Math Function1 : Math  Operator=transpose  SaturateOnIntegerOverflow=on
  Sqrt : Sqrt  SaturateOnIntegerOverflow=on
  Norm : Outport
  wires:
  Vec/1 -> Math Function1/1, Dot Product1/1
  Dot Product1/1 -> Sqrt/1
  Math Function1/1 -> Dot Product1/2
  Sqrt/1 -> Norm/1

== system cf_compare_model/PID_Estimator/AddNoise1 ==
  Signal : Inport
  Add2 : Sum
  Band-Limited White Noise : simulink/Sources/Band-Limited White Noise  Cov=est.noise_power  Ts=est.noise_sample_time  seed=rng_seed
  +Noise : Outport
  wires:
  Add2/1 -> +Noise/1
  Signal/1 -> Add2/1
  Band-Limited White Noise/1 -> Add2/2

== system cf_compare_model/PID_Estimator/AddNoise2 ==
  Signal : Inport
  Add2 : Sum
  Band-Limited White Noise : simulink/Sources/Band-Limited White Noise  Cov=est.noise_power  Ts=est.noise_sample_time  seed=rng_seed
  +Noise : Outport
  wires:
  Add2/1 -> +Noise/1
  Signal/1 -> Add2/1
  Band-Limited White Noise/1 -> Add2/2

== system cf_compare_model/PID_Estimator/AddNoise3 ==
  Signal : Inport
  Add2 : Sum
  Band-Limited White Noise : simulink/Sources/Band-Limited White Noise  Cov=est.noise_power  Ts=est.noise_sample_time  seed=rng_seed
  +Noise : Outport
  wires:
  Add2/1 -> +Noise/1
  Signal/1 -> Add2/1
  Band-Limited White Noise/1 -> Add2/2

== system cf_compare_model/PID_Estimator/Mahony ==
  A : Inport  PortDimensions=[1 3]
  ω : Inport  Port=2  PortDimensions=[1 3]
  rpy_quaternion : Inport  Port=3
  q : Inport  Port=4  PortDimensions=[1 4]
  Acceleration Error Estimate : Scope  Commented=on
  Add : Sum  Inputs=+++
  Add1 : Sum
  Constant : Constant  Value=0
  Cross Product : vrlib/Utilities/Cross Product
  Cross Product1 : vrlib/Utilities/Cross Product
  Gain1 : Gain  Gain=0.5
  Integrator : Integrator
  Integrator1 : Integrator  InitialCondition=[1,0,0,0]
  Ki : Gain  Gain=est.Ki
  Kp : Gain  Gain=est.Kp
  Mux : Mux  Inputs=2
  Normalize Vector : vrlib/Utilities/Normalize Vector  maxzero=.01
  Normalize Vector1 : vrlib/Utilities/Normalize Vector  maxzero=10e-4
  Total Error Estimate : Scope  Commented=on
  calc v : MATLAB Function  TreatAsAtomicUnit=on
  calc v3 : MATLAB Function  TreatAsAtomicUnit=on
  quatprod : MATLAB Function  TreatAsAtomicUnit=on
  Quaternion : Outport
  wires:
  ω/1 -> Add/3
  Normalize Vector/1 -> Cross Product/2
  calc v3/1(v) -> Cross Product1/1
  Cross Product1/1 -> Add1/1
  rpy_quaternion/1 -> calc v3/1(q)
  Cross Product/1 -> Add1/2, Acceleration Error Estimate/1
  q/1 -> quatprod/1(a), calc v/1(q)
  Normalize Vector1/1 -> Quaternion/1
  Integrator1/1 -> Normalize Vector1/1
  Integrator/1 -> Ki/1
  Mux/1 -> quatprod/2(b)
  quatprod/1(ab) -> Gain1/1
  Gain1/1 -> Integrator1/1
  Kp/1 -> Add/1
  Add/1 -> Mux/2
  calc v/1(v) -> Cross Product1/2, Cross Product/1
  Ki/1 -> Add/2
  Add1/1 -> Total Error Estimate/1, Kp/1, Integrator/1
  Constant/1 -> Mux/1
  A/1 -> Normalize Vector/1
